simulink model "Part_5"  (R2024a)
settings: Solver=VariableStepAuto  StartTime=0.0  StopTime=10.0  RelTol=1e-3
settings Model: Creator=HP  LastModifiedBy=sujay

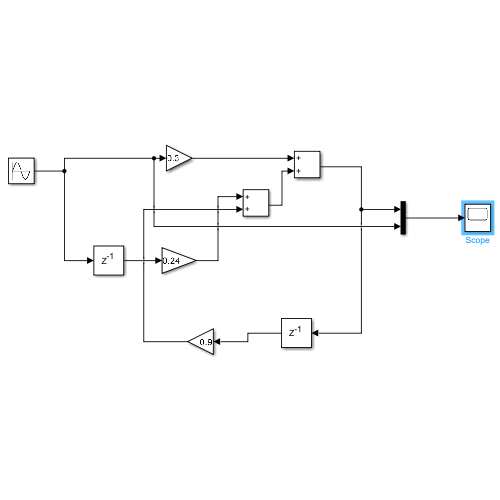
[thumbnail: Simulink's stored preview of the top-level diagram]
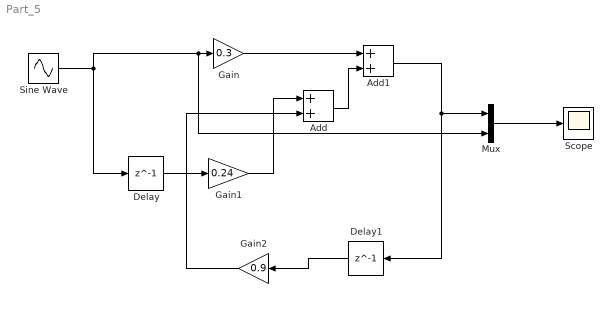
== system Part_5 ==
  Add : Sum
  Add1 : Sum
  Delay : Delay  DelayLength=1  InitialCondition=0
  Delay1 : Delay  DelayLength=1  InitialCondition=0
  Gain : Gain  Gain=0.3
  Gain1 : Gain  Gain=0.24
  Gain2 : Gain  Gain=0.9
  Mux : Mux  Inputs=2
  Scope : Scope
  Sine Wave : Sin  SampleTime=0
  wires:
  Sine Wave/1 -> Delay/1, Mux/2, Gain/1
  Gain/1 -> Add1/1
  Add/1 -> Add1/2
  Gain1/1 -> Add/1
  Delay/1 -> Gain1/1
  Gain2/1 -> Add/2
  Delay1/1 -> Gain2/1
  Add1/1 -> Delay1/1, Mux/1
  Mux/1 -> Scope/1
